simulink model "Linearity_Test1"  (R2018b)
settings: Solver=VariableStepAuto  StartTime=0.0  StopTime=10.0  RelTol=1e-3
settings Model: Creator=hp  LastModifiedBy=hp

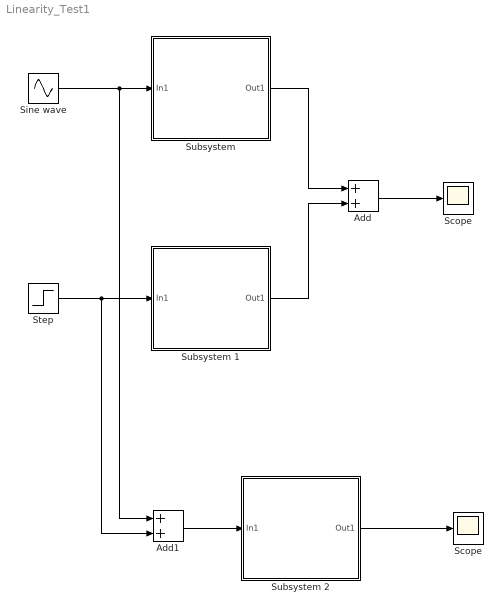
== system Linearity_Test1 ==
  Add : Sum
  Add1 : Sum
  Scope : Scope
  "Scope " : Scope
  Sine wave : Sin  SampleTime=0
  Step : Step  SampleTime=0
  "Subsystem " : Subsystem
  Subsystem 1 : Subsystem
  Subsystem 2 : Subsystem
  wires:
  Sine wave/1 -> Add1/1, "Subsystem "/1(In1)
  Step/1 -> Add1/2, Subsystem 1/1(In1)
  Subsystem 1/1(Out1) -> Add/2
  "Subsystem "/1(Out1) -> Add/1
  Add/1 -> "Scope "/1
  Add1/1 -> Subsystem 2/1(In1)
  Subsystem 2/1(Out1) -> Scope/1

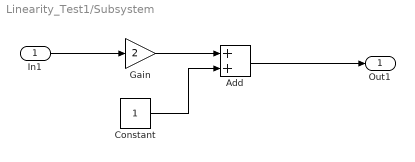
== system Linearity_Test1/Subsystem  ==
  In1 : Inport
  "Add " : Sum
  "Constant " : Constant
  "Gain " : Gain  Gain=2
  Out1 : Outport
  wires:
  "Constant "/1 -> "Add "/2
  "Add "/1 -> Out1/1
  In1/1 -> "Gain "/1
  "Gain "/1 -> "Add "/1

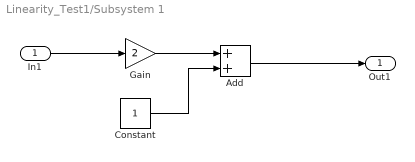
== system Linearity_Test1/Subsystem 1 ==
  In1 : Inport
  "Add " : Sum
  "Constant " : Constant
  "Gain " : Gain  Gain=2
  Out1 : Outport
  wires:
  "Constant "/1 -> "Add "/2
  "Add "/1 -> Out1/1
  In1/1 -> "Gain "/1
  "Gain "/1 -> "Add "/1

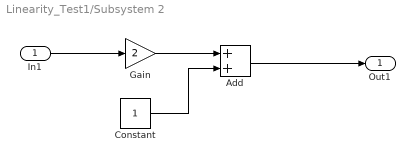
== system Linearity_Test1/Subsystem 2 ==
  In1 : Inport
  "Add " : Sum
  "Constant " : Constant
  "Gain " : Gain  Gain=2
  Out1 : Outport
  wires:
  "Constant "/1 -> "Add "/2
  "Add "/1 -> Out1/1
  In1/1 -> "Gain "/1
  "Gain "/1 -> "Add "/1
